simulink model "lvlh_control_sim"  (R2023b)
settings: Solver=ode5  StartTime=0.0  StopTime=100  RelTol=1e-3
values from neighbouring files (symbols this model uses):
  A = [ ... (first row only)    [complete_model.m]    (also in control_lvlh.m; lvlh_control.m = zeros(6,6); untitled.m = zeros(6,6))
  a = 6.851221970532768e+03    (= 6851.22197053)    [complete_model.m]    (also in control_lvlh.m; lvlh_control.m; untitled.m)
  alpha1 = 0.4    [complete_model.m]    (also in control_lvlh.m; lvlh_control.m; untitled.m)
  alpha2 = 0.1    [complete_model.m]    (also in control_lvlh.m; lvlh_control.m; untitled.m)
  alpha3 = 0.5    [complete_model.m]    (also in control_lvlh.m; lvlh_control.m; untitled.m)
  B = [ ... (first row only)    [complete_model.m]    (also in control_lvlh.m; lvlh_control.m = zeros(6,3); untitled.m = zeros(6,3))
  C = [ ... (first row only)    [complete_model.m]    (also in control_lvlh.m; lvlh_control.m = [[0 0 0 1 0 0];[0 0 0 0 1 0]; [0 0 0 0 0 1]]; untitled.m = [[0 0 0 1 0 0];[0 0 0 0 1 0]; [0 0 0 0 0 1]])
  D = zeros(3)    [complete_model.m]    (also in control_lvlh.m; lvlh_control.m = zeros(3,3); untitled.m = zeros(3,3))
  e = 0    [complete_model.m]    (also in control_lvlh.m; lvlh_control.m; untitled.m)
  FOV_earth = deg2rad(33)    [complete_model.m]    (also in control_lvlh.m; lvlh_control.m; untitled.m)
  FOV_sun = deg2rad(85)    [control_lvlh.m]    (also in lvlh_control.m; untitled.m)
  freq_earth = 30    [complete_model.m]    (also in control_lvlh.m = 5; lvlh_control.m = 5; untitled.m = 5)
  freq_mag = 30    [complete_model.m]    (also in control_lvlh.m = 5; lvlh_control.m = 5; untitled.m = 5)
  freq_sun = 30    [complete_model.m]    (also in control_lvlh.m = 5; lvlh_control.m = 5; untitled.m = 5)
  H0 = sqrt(g01^2+g11^2+h11^2)*1e-9    [complete_model.m]    (also in control_lvlh.m; lvlh_control.m; untitled.m)
  I = diag([I1 I2 I3])    [complete_model.m]    (also in control_lvlh.m; lvlh_control.m; untitled.m)
  Iinv = I\eye(3)    [complete_model.m]    (also in control_lvlh.m; lvlh_control.m; untitled.m)
  incl = deg2rad(11.5)    [complete_model.m]    (also in control_lvlh.m; lvlh_control.m; untitled.m)
  jb = [0.01; 0.05; 0.01]    [complete_model.m]    (also in control_lvlh.m; lvlh_control.m; untitled.m)
  K = place(A,B,p)    [complete_model.m]    (also in control_lvlh.m = [Kd Kp]; lvlh_control.m = 1/100*K)
  L = Ltr'    [lvlh_control.m]    (also in untitled.m)
  n = sqrt(mu/a^3)    [complete_model.m]    (also in control_lvlh.m; lvlh_control.m; untitled.m)
  omega0 = 0.06 * rand(3,1)    [complete_model.m]    (also in control_lvlh.m = [0; 0; n]; lvlh_control.m = [0; 0; n]; untitled.m = [0; 0; n])
  omegaE = deg2rad(15)/3600    [complete_model.m]    (also in control_lvlh.m; lvlh_control.m; untitled.m)
  rs = -rr    [complete_model.m]    (also in control_lvlh.m; lvlh_control.m; untitled.m)
  Rt = astroConstants(23)    [complete_model.m]    (also in control_lvlh.m; lvlh_control.m; untitled.m)
  s0 = 2*pi*rand(3,1)    [complete_model.m]    (also in control_lvlh.m = [2.099, -0.2003, -1.703]; lvlh_control.m = [2.099, -0.2003, -1.703]; untitled.m = [2.099, -0.2003, -1.703])
  tol = 0.2    [complete_model.m]    (also in control_lvlh.m; lvlh_control.m; untitled.m)
  variance_E_sens = (deg2rad(0.05)/3)^2    [lvlh_control.m]    (also in untitled.m)
undefined symbols (not defined in the file or in its folder): magnitude
libraries: vrlib x8, matrix_library x6, simulink x6, sharedutil x2, dspmathops x2, dspfactors x1, simulink_extras x1
(part 1 of 2)
settings Model: Creator=danie  LastModifiedBy=danie

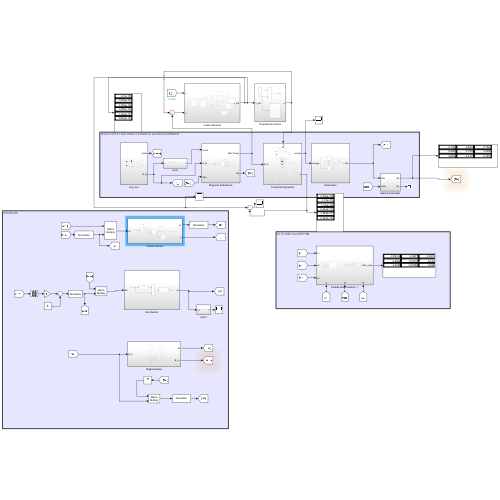
[thumbnail: Simulink's stored preview of the top-level diagram]
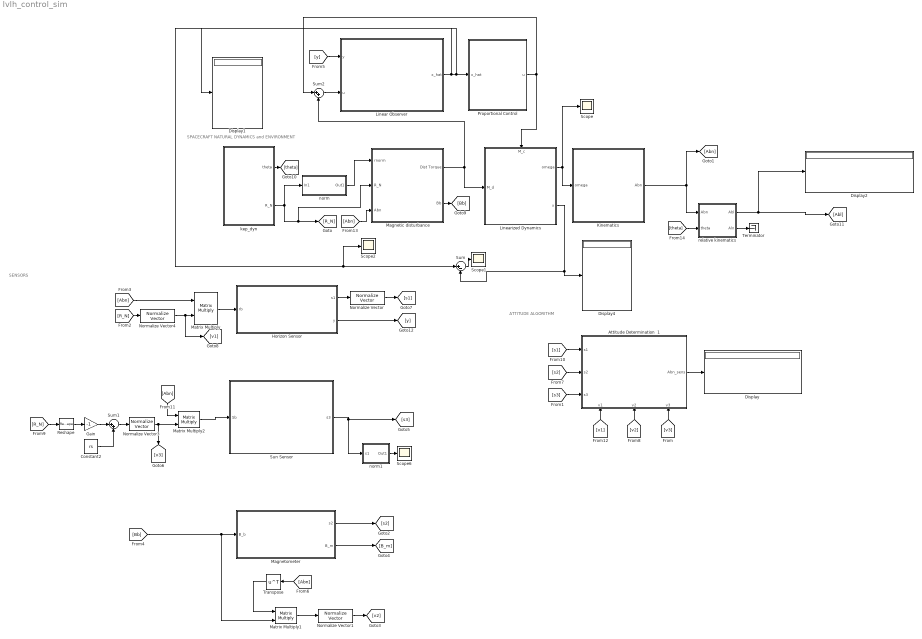
== system lvlh_control_sim ==
  note: SENSORS
  note: ATTITUDE ALGORITHM
  note: SPACECRAFT NATURAL DYNAMICS and ENVIRONMENT
  Attitude Determination  1 : Subsystem
      settings: PortSchema="{\"entries\":[{\"content\":{\"sides\":[{\"content\":{\"connectorIds\":[\"In1\",\"In2\",\"In3\"]},\"type\":\"ConnectorPlacement.EquallySpacedRectSide\",\"uuid\":\"730966cf-d0d7-44a0-92f0-b5324480e7cc\"},{\"content\":{\"connectorIds\":[\"Out1\"],\"side\":\"RIGHT\"},\"type\":\"ConnectorPlacement.EquallySpacedRectSide\",\"uuid\":\"c83e6b57-46fe-4a45-9824-d3495e15bf6a\"},{\"content\":{\"side\":\"TOP\"},\"type\":\"ConnectorPlacement.EquallySpacedRectSide\",\"uuid\":\"4938c298-c2b3-45b7-bcb0-70b8132dabc6\"},{\"content\":{\"connectorIds\":[\"In4\",\"In5\",\"In6\"],\"side\":\"BOTTOM\"},\"type\":\"ConnectorPlacement.EquallySpacedRectSide\",\"uuid\":\"6d6a244e-80db-423b-a0a5-9a5face48fcb\"}]},\"type\":\"ConnectorPlacement.EquallySpacedConnector\",\"uuid\":\"7eb6767d-3ff0-4577-86c9-ebc5e763f220\"}],\"packageUris\":[\"http://schema.mathworks.com/mf0/Connector/R2020b\"],\"version\":\"1.0\"}"
  Constant2 : Constant  Value=rs
  Display{,1..2,4} (4 alike) : Display
  Gain : Gain  Gain=-1
  Horizon Sensor : Subsystem
  Kinematics : Subsystem
  Linear Observer : Subsystem
  Linearized Dynamics : Subsystem
      settings: PortSchema="{\"entries\":[{\"content\":{\"sides\":[{\"content\":{\"connectorIds\":[\"In1\"]},\"type\":\"ConnectorPlacement.EquallySpacedRectSide\",\"uuid\":\"c1c0c392-5a65-42dc-acc1-f79aac47fb4a\"},{\"content\":{\"connectorIds\":[\"Out1\",\"Out2\"],\"side\":\"RIGHT\"},\"type\":\"ConnectorPlacement.EquallySpacedRectSide\",\"uuid\":\"022a04b8-112e-4b43-aa4b-234ec6f248c8\"},{\"content\":{\"connectorIds\":[\"In2\"],\"side\":\"TOP\"},\"type\":\"ConnectorPlacement.EquallySpacedRectSide\",\"uuid\":\"afc410f0-4ae5-435d-a431-df883452497d\"}]},\"type\":\"ConnectorPlacement.EquallySpacedConnector\",\"uuid\":\"3545f0ca-e723-442b-9659-f094d9054fb0\"}],\"packageUris\":[\"http://schema.mathworks.com/mf0/Connector/R2020b\"],\"version\":\"1.0\"}"
  Magnetic disturbance : Subsystem
  Magnetometer : Subsystem
  Matrix Multiply : Product  Multiplication=Matrix(*)
  Matrix Multiply1 : Product  Multiplication=Matrix(*)
  Matrix Multiply2 : Product  Multiplication=Matrix(*)
  Normalize Vector{,1,3..4} (4 alike) : vrlib/Utilities/Normalize Vector  maxzero=0
  Proportional Control : Subsystem
  Reshape : Reshape  OutputDimensionality=Column vector (2-D)
  Scope{,1..2,6} (4 alike) : Scope
  Sum : Sum  Inputs=|+-
  Sum1 : Sum  Inputs=|++
  Sum2 : Sum  Inputs=|++
  Sun Sensor : Subsystem
  Terminator : Terminator
  Transpose : Math  Operator=transpose
  kep_dyn : Subsystem
  norm : Subsystem
  norm1 : Subsystem
  relative kinematics : Subsystem
  wires:
  Kinematics/1(Abn) -> relative kinematics/1(Abn), [Abn]
  [v1] -> Attitude Determination  1/4(v1)
  [Abn] -> Matrix Multiply2/1
  [theta] -> relative kinematics/2(theta)
  Matrix Multiply/1 -> Horizon Sensor/1(rb)
  relative kinematics/1(Abl) -> Display2/1, [Abl]
  Matrix Multiply1/1 -> Normalize Vector1/1
  norm/1(Out1) -> Magnetic disturbance/1(rnorm)
  Normalize Vector1/1 -> [v2]
  [s2] -> Attitude Determination  1/2(s2)
  Constant2/1 -> Sum1/2
  Sum1/1 -> Normalize Vector3/1
  Normalize Vector/1 -> [s1]
  [s1] -> Attitude Determination  1/1(s1)
  kep_dyn/1(theta) -> [theta]
  kep_dyn/2(R_N) -> Magnetic disturbance/2(R_N), [R_N], norm/1(In1)
  [s3] -> Attitude Determination  1/3(s3)
  Magnetometer/2("B_m ") -> [B_m]
  [Abn] -> Transpose/1
  Magnetic disturbance/2(Bb) -> [Bb]
  [Abn] -> Magnetic disturbance/3(Abn)
  Horizon Sensor/1(s1) -> Normalize Vector/1
  [R_N] -> Normalize Vector4/1
  [Bb] -> Matrix Multiply1/2, Magnetometer/1(B_b)
  Sun Sensor/1(s3) -> norm1/1(s1), [s3]
  [R_N] -> Reshape/1
  Matrix Multiply2/1 -> Sun Sensor/1(Sb)
  Transpose/1 -> Matrix Multiply1/1
  Normalize Vector4/1 -> [v1], Matrix Multiply/2
  norm1/1(Out1) -> Scope6/1
  Attitude Determination  1/1(Abn_sens) -> Display/1
  Normalize Vector3/1 -> Matrix Multiply2/2, [v3]
  Magnetometer/1(s2) -> [s2]
  [v3] -> Attitude Determination  1/6(v3)
  relative kinematics/2(Aln) -> Terminator/1
  [Abn] -> Matrix Multiply/1
  Gain/1 -> Sum1/1
  [v2] -> Attitude Determination  1/5(v2)
  Reshape/1 -> Gain/1
  Magnetic disturbance/1(Dist Torque) -> Sum2/2, Linearized Dynamics/1(M_d)
  Linearized Dynamics/1(omega) -> Kinematics/1(omega), Scope/1
  Horizon Sensor/2(y) -> [y]
  [y] -> Linear Observer/1(y)
  Linearized Dynamics/2(x) -> Sum/2, Display4/1
  Sum/1 -> Scope1/1
  Linear Observer/1(x_hat) -> Display1/1, Scope2/1, Sum/1, Proportional Control/1(x_hat)
  Sum2/1 -> Linear Observer/2(u)
  Proportional Control/1(u) -> Linearized Dynamics/2(M_c), Sum2/1

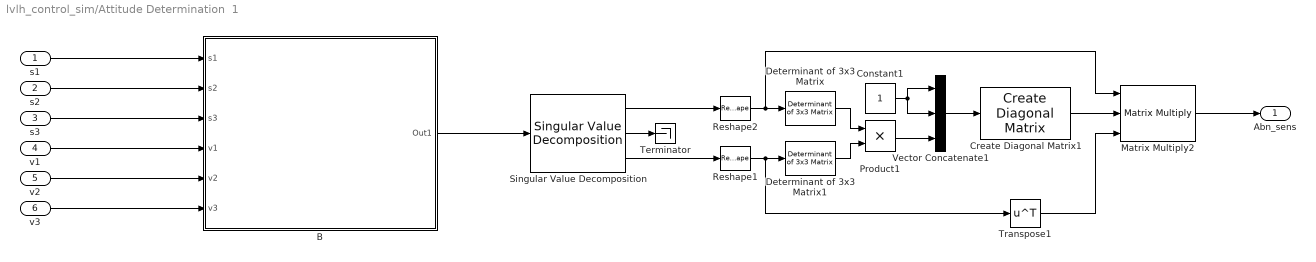
== system lvlh_control_sim/Attitude Determination  1 ==
  s1 : Inport
  s2 : Inport  Port=2
  s3 : Inport  Port=3
  v1 : Inport  Port=4
  v2 : Inport  Port=5
  v3 : Inport  Port=6
  B : Subsystem
  Constant1 : Constant
  Create Diagonal Matrix1 : matrix_library/Create Diagonal Matrix
      settings: LibrarySourceBlock=|
      | simulink/Matrix
      | Operations/Create Diagonal
      | Matrix
  Determinant of 3x3 Matrix : sharedutil/Determinant of 3x3 Matrix  aMode=aMode
      settings: LibrarySourceBlock=|
      | aerolibutil/Determinant of
      | 3x3 Matrix
  Determinant of 3x3 Matrix1 : sharedutil/Determinant of 3x3 Matrix  aMode=aMode
      settings: LibrarySourceBlock=|
      | aerolibutil/Determinant of
      | 3x3 Matrix
  Matrix Multiply2 : Product  Inputs=3  Multiplication=Matrix(*)
  Product1 : Product
  Reshape1 : Reshape  OutputDimensionality=Customize  OutputDimensions=[3,3]
  Reshape2 : Reshape  OutputDimensionality=Customize  OutputDimensions=[3,3]
  Singular Value Decomposition : dspfactors/Singular Value Decomposition  wantv=on  wanterr=off  SimulateUsing=Interpreted execution
  Terminator : Terminator
  Transpose1 : Math  Operator=transpose
  Vector Concatenate1 : Concatenate  NumInputs=3
  Abn_sens : Outport
  wires:
  Reshape1/1 -> Transpose1/1, Determinant of 3x3 Matrix1/1
  Singular Value Decomposition/3 -> Reshape1/1
  Singular Value Decomposition/1 -> Reshape2/1
  Reshape2/1 -> Determinant of 3x3 Matrix/1, Matrix Multiply2/1
  Determinant of 3x3 Matrix1/1 -> Product1/2
  Determinant of 3x3 Matrix/1 -> Product1/1
  Product1/1 -> Vector Concatenate1/3
  Constant1/1 -> Vector Concatenate1/2, Vector Concatenate1/1
  Vector Concatenate1/1 -> Create Diagonal Matrix1/1
  Create Diagonal Matrix1/1 -> Matrix Multiply2/2
  Transpose1/1 -> Matrix Multiply2/3
  s1/1 -> B/1(s1)
  s2/1 -> B/2(s2)
  s3/1 -> B/3(s3)
  v1/1 -> B/4(v1)
  v2/1 -> B/5(v2)
  v3/1 -> B/6(v3)
  B/1(Out1) -> Singular Value Decomposition/1
  Matrix Multiply2/1 -> Abn_sens/1
  Singular Value Decomposition/2 -> Terminator/1

== system lvlh_control_sim/Horizon Sensor ==
  rb : Inport
  Constant : Constant
  Display : Display
  Display1 : Display
  EH sensor modeling : Subsystem
  FOV CHECK : Subsystem  Commented=on
  Gain : Gain  Gain=-1
  Product1 : Product
  s1 : Outport
  y : Outport  Port=2
  wires:
  rb/1 -> Gain/1
  Product1/1 -> EH sensor modeling/1(rb)
  EH sensor modeling/1(q) -> s1/1  "direction of earth"
  EH sensor modeling/2(y) -> y/1, Display/1
  Gain/1 -> FOV CHECK/1(In1), Display1/1, Product1/2
  Constant/1 -> Product1/1

== system lvlh_control_sim/Kinematics ==
  omega : Inport
  Kinematics 312 : Subsystem
  Kinematics 313 : Subsystem
  Merge : Merge
  NOT : Logic  Operator=NOT  IconShape=distinctive  AllPortsSameDT=off  OutDataTypeStr=boolean
  System switcher : Subsystem
  To Workspace : ToWorkspace  VariableName=A  SaveFormat=Timeseries  SampleTime=-1
  Abn : Outport
  wires:
  NOT/1 -> Kinematics 313/Enable
  omega/1 -> Kinematics 312/1(w), Kinematics 313/1(w)
  System switcher/1(flag) -> Kinematics 312/Enable, NOT/1
  Kinematics 313/1(A) -> Merge/2
  Merge/1 -> Abn/1, To Workspace/1  "A"
  Kinematics 312/1(A) -> Merge/1

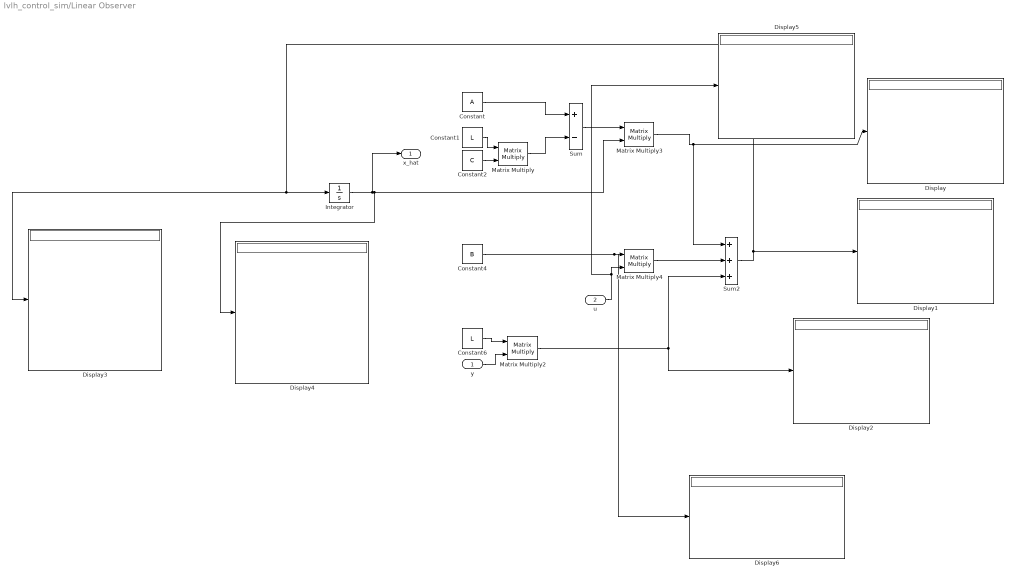
== system lvlh_control_sim/Linear Observer ==
  y : Inport
  u : Inport  Port=2
  Constant : Constant  Value=A
  Constant1 : Constant  Value=L
  Constant2 : Constant  Value=C
  Constant4 : Constant  Value=B
  Constant6 : Constant  Value=L
  Display{,1..6} (7 alike) : Display
  Integrator : Integrator  InitialCondition=[0;0;0;0;0;0]
  Matrix Multiply{,2..4} (4 alike) : Product  Multiplication=Matrix(*)
  Sum : Sum  Inputs=+-
  Sum2 : Sum  Inputs=+++
  x_hat : Outport
  wires:
  Constant1/1 -> Matrix Multiply/1
  Constant2/1 -> Matrix Multiply/2
  Matrix Multiply/1 -> Sum/2
  Constant/1 -> Sum/1
  Constant6/1 -> Matrix Multiply2/1
  y/1 -> Matrix Multiply2/2
  u/1 -> Matrix Multiply4/2, Display5/1
  Constant4/1 -> Display6/1, Matrix Multiply4/1
  Sum/1 -> Matrix Multiply3/1
  Matrix Multiply4/1 -> Sum2/2
  Matrix Multiply2/1 -> Sum2/3, Display2/1
  Matrix Multiply3/1 -> Display/1, Sum2/1
  Sum2/1 -> Integrator/1, Display3/1, Display1/1
  Integrator/1 -> Display4/1, Matrix Multiply3/2, x_hat/1

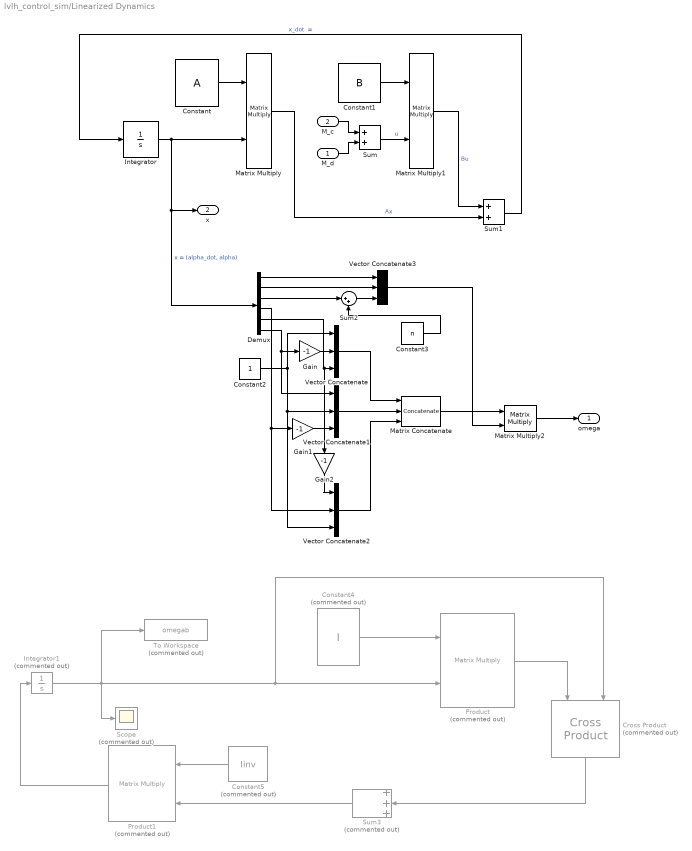
== system lvlh_control_sim/Linearized Dynamics ==
  M_d : Inport
  M_c : Inport  Port=2
  Constant : Constant  Value=A
  Constant1 : Constant  Value=B
  Constant2 : Constant
  Constant3 : Constant  Value=n
  Constant4 : Constant  Commented=on  Value=I
  Constant5 : Constant  Commented=on  Value=Iinv
  Cross Product : matrix_library/Cross Product  Commented=on
  Demux : Demux  Outputs=6
  Gain : Gain  Gain=-1
  Gain1 : Gain  Gain=-1
  Gain2 : Gain  Gain=-1
  Integrator : Integrator  InitialCondition=[1e-6; 1e-6; n; 0;0;0]
  Integrator1 : Integrator  Commented=on  InitialCondition=omega0
  Matrix Concatenate : Concatenate  NumInputs=3  Mode=Multidimensional array  ConcatenateDimension=2
  Matrix Multiply : Product  Multiplication=Matrix(*)
  Matrix Multiply1 : Product  Multiplication=Matrix(*)
  Matrix Multiply2 : Product  Multiplication=Matrix(*)
  Product : Product  Commented=on  Multiplication=Matrix(*)
  Product1 : Product  Commented=on  Multiplication=Matrix(*)
  Scope : Scope  Commented=on
  Sum : Sum
  Sum1 : Sum
  Sum2 : Sum  Inputs=|++
  Sum3 : Sum  Commented=on  Inputs=+++
  To Workspace : ToWorkspace  Commented=on  VariableName=omegab  SampleTime=-1
  Vector Concatenate{,1..3} (4 alike) : Concatenate  NumInputs=3
  omega : Outport
  x : Outport  Port=2
  wires:
  Integrator/1 -> x/1, Demux/1, Matrix Multiply/2  "x = (alpha_dot, alpha)"
  Constant/1 -> Matrix Multiply/1
  Constant1/1 -> Matrix Multiply1/1
  Sum/1 -> Matrix Multiply1/2  "u"
  M_c/1 -> Sum/1
  Matrix Multiply1/1 -> Sum1/1  "Bu"
  Matrix Multiply/1 -> Sum1/2  "Ax"
  Sum1/1 -> Integrator/1  "x_dot  ="
  Constant2/1 -> Vector Concatenate/1, Vector Concatenate2/3, Vector Concatenate1/2
  Demux/6 -> Vector Concatenate1/1, Gain/1
  Gain/1 -> Vector Concatenate/2
  Demux/5 -> Vector Concatenate/3, Gain2/1
  Demux/4 -> Vector Concatenate2/2, Gain1/1
  Gain1/1 -> Vector Concatenate1/3
  Gain2/1 -> Vector Concatenate2/1
  Vector Concatenate/1 -> Matrix Concatenate/1
  Vector Concatenate1/1 -> Matrix Concatenate/2
  Vector Concatenate2/1 -> Matrix Concatenate/3
  Matrix Concatenate/1 -> Matrix Multiply2/1
  Demux/1 -> Vector Concatenate3/1
  Demux/2 -> Vector Concatenate3/2
  Demux/3 -> Sum2/1
  Constant3/1 -> Sum2/2
  Sum2/1 -> Vector Concatenate3/3
  Vector Concatenate3/1 -> Matrix Multiply2/2
  Matrix Multiply2/1 -> omega/1
  Sum3/1 -> Product1/2
  Constant4/1 -> Product/1
  Constant5/1 -> Product1/1
  Cross Product/1 -> Sum3/2
  Integrator1/1 -> To Workspace/1, Scope/1, Product/2, Cross Product/2
  Product/1 -> Cross Product/1
  Product1/1 -> Integrator1/1
  M_d/1 -> Sum/2

== system lvlh_control_sim/Magnetic disturbance ==
  rnorm : Inport
  R_N : Inport  Port=2
  Abn : Inport  Port=3
  "Magnetic Torque " : Subsystem
  Matrix Multiply : Product  Multiplication=Matrix(*)
  Normalize Vector : vrlib/Utilities/Normalize Vector  maxzero=0
  Scope : Scope
  Scope1 : Scope
  To Workspace1 : ToWorkspace  VariableName=mag_torque  SampleTime=-1
  Dist Torque : Outport
  Bb : Outport  Port=2
  wires:
  rnorm/1 -> "Magnetic Torque "/1(rnorm)
  Abn/1 -> Matrix Multiply/1, "Magnetic Torque "/2(Abn)
  "Magnetic Torque "/1(M_mag) -> To Workspace1/1, Scope1/1, Dist Torque/1
  "Magnetic Torque "/2(Bb) -> Scope/1, Bb/1
  R_N/1 -> Normalize Vector/1
  Matrix Multiply/1 -> "Magnetic Torque "/3(rb)
  Normalize Vector/1 -> Matrix Multiply/2

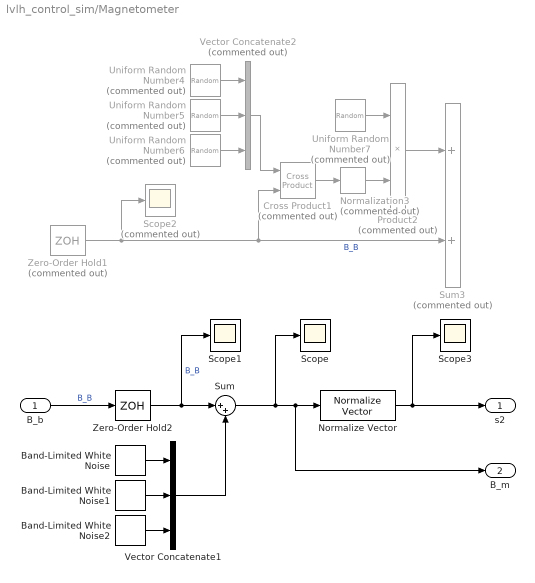
== system lvlh_control_sim/Magnetometer ==
  B_b : Inport
  Band-Limited White Noise : simulink/Sources/Band-Limited White Noise  Cov=[1.18^2 *1e-18]  Ts=1/freq_mag  seed=[23341]
  Band-Limited White Noise1 : simulink/Sources/Band-Limited White Noise  Cov=[1.18^2 *1e-18]  Ts=1/freq_mag  seed=[23341]
  Band-Limited White Noise2 : simulink/Sources/Band-Limited White Noise  Cov=[1.18^2 *1e-18]  Ts=1/freq_mag  seed=[23341]
  Cross Product1 : matrix_library/Cross Product  Commented=on
  Normalization3 : dspmathops/Normalization  Commented=on  NormType=2-norm  Bias=1e-10  NormOver=Each column  Dimension=1  roundingMode=Floor  overflowMode=off  accumDataTypeStr=Inherit: Same as product output  accumLastDataTypeStr=Inherit: Same as product output  outputDataTypeStr=Inherit: Same as product output  outputMin=[]  outputMax=[]  outputLastDataTypeStr=Inherit: Same as product output
  Normalize Vector : vrlib/Utilities/Normalize Vector  maxzero=0
  Product2 : Product  Commented=on
  Scope : Scope
  Scope1 : Scope
  Scope2 : Scope  Commented=on
  Scope3 : Scope
  Sum : Sum  Inputs=|++
  Sum3 : Sum  Commented=on
  Uniform Random Number4 : UniformRandomNumber  Commented=on  SampleTime=1/30
  Uniform Random Number5 : UniformRandomNumber  Commented=on  SampleTime=1/30
  Uniform Random Number6 : UniformRandomNumber  Commented=on  SampleTime=1/30
  Uniform Random Number7 : UniformRandomNumber  Commented=on  Minimum=0  Maximum=tan(deg2rad(0.5))  SampleTime=1/30
  Vector Concatenate1 : Concatenate  NumInputs=3
  Vector Concatenate2 : Concatenate  Commented=on  NumInputs=3
  Zero-Order Hold1 : ZeroOrderHold  Commented=on  SampleTime=1/30
  Zero-Order Hold2 : ZeroOrderHold  SampleTime=1/freq_mag
  s2 : Outport
  "B_m " : Outport  Port=2
  wires:
  Zero-Order Hold1/1 -> Cross Product1/2, Sum3/2, Scope2/1  "B_B"
  Product2/1 -> Sum3/1
  Normalization3/1 -> Product2/2
  Uniform Random Number4/1 -> Vector Concatenate2/1
  Uniform Random Number6/1 -> Vector Concatenate2/3
  Vector Concatenate2/1 -> Cross Product1/1
  Cross Product1/1 -> Normalization3/1
  Uniform Random Number5/1 -> Vector Concatenate2/2
  Uniform Random Number7/1 -> Product2/1
  B_b/1 -> Zero-Order Hold2/1  "B_B"
  Zero-Order Hold2/1 -> Scope1/1, Sum/1  "B_B"
  Band-Limited White Noise2/1 -> Vector Concatenate1/3
  Band-Limited White Noise1/1 -> Vector Concatenate1/2
  Band-Limited White Noise/1 -> Vector Concatenate1/1
  Normalize Vector/1 -> Scope3/1, s2/1
  Vector Concatenate1/1 -> Sum/2
  Sum/1 -> Scope/1, "B_m "/1, Normalize Vector/1

== system lvlh_control_sim/Proportional Control ==
  x_hat : Inport
  Constant : Constant  Value=-K
  Display : Display
  Matrix Multiply : Product  Multiplication=Matrix(*)
  u : Outport
  wires:
  x_hat/1 -> Display/1, Matrix Multiply/2
  Constant/1 -> Matrix Multiply/1
  Matrix Multiply/1 -> u/1

== system lvlh_control_sim/Sun Sensor ==
  Sb : Inport
  FOV CHECK : Subsystem
  Product : Product
  Sun Sensor Modeling : Subsystem
  s3 : Outport
  wires:
  Sb/1 -> Product/2, FOV CHECK/1(In1)  "Sb"
  Sun Sensor Modeling/1(s3) -> s3/1
  Product/1 -> Sun Sensor Modeling/1(Sb)  "Sb"
  FOV CHECK/1(b) -> Product/1

== system lvlh_control_sim/kep_dyn ==
  A_np : Constant  Value=A_pn'
  Constant : Constant  Value=0
  Constant1 : Constant  Value=e
  Cos : Trigonometry  Operator=cos
  Integrator : Integrator
  Matrix Multiply : Product  Multiplication=Matrix(*)
  Product2 : Product
  Sin : Trigonometry
  Vector Concatenate : Concatenate  NumInputs=3
  r_norm : Subsystem
  theta integration : Subsystem
      settings: PortSchema="{\"entries\":[{\"content\":{\"sides\":[{\"content\":{\"connectorIds\":[\"In1\"]},\"type\":\"ConnectorPlacement.EquallySpacedRectSide\",\"uuid\":\"3f1b1ec9-07ed-4eb1-9e41-630dc5613e97\"},{\"content\":{\"connectorIds\":[\"Out1\",\"In2\"],\"side\":\"RIGHT\"},\"type\":\"ConnectorPlacement.EquallySpacedRectSide\",\"uuid\":\"22d0f7bc-714c-4365-a26c-07047ff4be14\"},{\"content\":{\"side\":\"TOP\"},\"type\":\"ConnectorPlacement.EquallySpacedRectSide\",\"uuid\":\"875f7006-d698-4730-93ae-1a7d05f24054\"}]},\"type\":\"ConnectorPlacement.EquallySpacedConnector\",\"uuid\":\"799b65b1-faea-432b-9f3f-2d21984184cd\"}],\"packageUris\":[\"http://schema.mathworks.com/mf0/Connector/R2020b\"],\"version\":\"1.0\"}"
  theta : Outport
  R_N : Outport  Port=2
  wires:
  Integrator/1 -> Sin/1, Cos/1, r_norm/2(theta), theta/1, theta integration/1(theta)
  theta integration/1(theta_dot) -> Integrator/1
  Constant/1 -> Vector Concatenate/3
  Cos/1 -> Vector Concatenate/1
  Constant1/1 -> r_norm/1(e), theta integration/2(e)
  r_norm/1(r) -> Product2/1
  Vector Concatenate/1 -> Product2/2
  Sin/1 -> Vector Concatenate/2
  A_np/1 -> Matrix Multiply/1
  Product2/1 -> Matrix Multiply/2
  Matrix Multiply/1 -> R_N/1

== system lvlh_control_sim/norm ==
  In1 : Inport
  Dot Product : DotProduct  OutDataTypeStr=Inherit: Inherit via internal rule
  Sqrt : Sqrt
  Out1 : Outport
  wires:
  In1/1 -> Dot Product/1, Dot Product/2
  Dot Product/1 -> Sqrt/1
  Sqrt/1 -> Out1/1

== system lvlh_control_sim/norm1 ==
  s1 : Inport
  Dot Product : DotProduct  OutDataTypeStr=Inherit: Inherit via internal rule
  Square Root : Sqrt
  Out1 : Outport
  wires:
  s1/1 -> Dot Product/1, Dot Product/2
  Dot Product/1 -> Square Root/1
  Square Root/1 -> Out1/1

== system lvlh_control_sim/relative kinematics ==
  Abn : Inport
  theta : Inport  Port=2
  Constant : Constant  Value=A_pn'
  Matrix Multiply : Product  Multiplication=Matrix(*)
  Matrix Multiply2 : Product  Multiplication=Matrix(*)
  Subsystem : Subsystem
  Transpose : Math  Operator=transpose
  Abl : Outport
  Aln : Outport  Port=2
  wires:
  Abn/1 -> Matrix Multiply2/1
  Matrix Multiply/1 -> Transpose/1, Matrix Multiply2/2  "A_nl"
  Matrix Multiply2/1 -> Abl/1
  theta/1 -> Subsystem/1(theta)
  Subsystem/1(A_PL) -> Matrix Multiply/2  "A_PL"
  Constant/1 -> Matrix Multiply/1  "A_np"
  Transpose/1 -> Aln/1

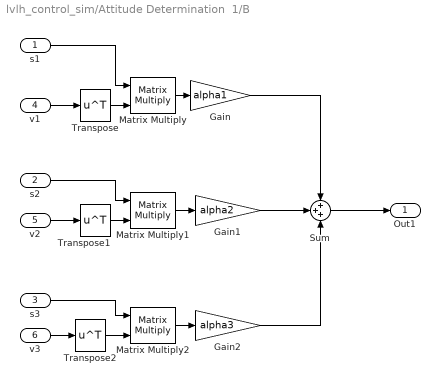
== system lvlh_control_sim/Attitude Determination  1/B ==
  s1 : Inport
  s2 : Inport  Port=2
  s3 : Inport  Port=3
  v1 : Inport  Port=4
  v2 : Inport  Port=5
  v3 : Inport  Port=6
  Gain : Gain  Gain=alpha1
  Gain1 : Gain  Gain=alpha2
  Gain2 : Gain  Gain=alpha3
  Matrix Multiply : Product  Multiplication=Matrix(*)
  Matrix Multiply1 : Product  Multiplication=Matrix(*)
  Matrix Multiply2 : Product  Multiplication=Matrix(*)
  Sum : Sum  Inputs=+++
  Transpose : Math  Operator=transpose
  Transpose1 : Math  Operator=transpose
  Transpose2 : Math  Operator=transpose
  Out1 : Outport
  wires:
  v1/1 -> Transpose/1
  Transpose/1 -> Matrix Multiply/2
  s1/1 -> Matrix Multiply/1
  Transpose1/1 -> Matrix Multiply1/2
  s2/1 -> Matrix Multiply1/1
  Transpose2/1 -> Matrix Multiply2/2
  v3/1 -> Transpose2/1
  Sum/1 -> Out1/1
  Matrix Multiply/1 -> Gain/1
  Matrix Multiply1/1 -> Gain1/1
  Matrix Multiply2/1 -> Gain2/1
  Gain/1 -> Sum/1
  Gain1/1 -> Sum/2
  Gain2/1 -> Sum/3
  v2/1 -> Transpose1/1
  s3/1 -> Matrix Multiply2/1

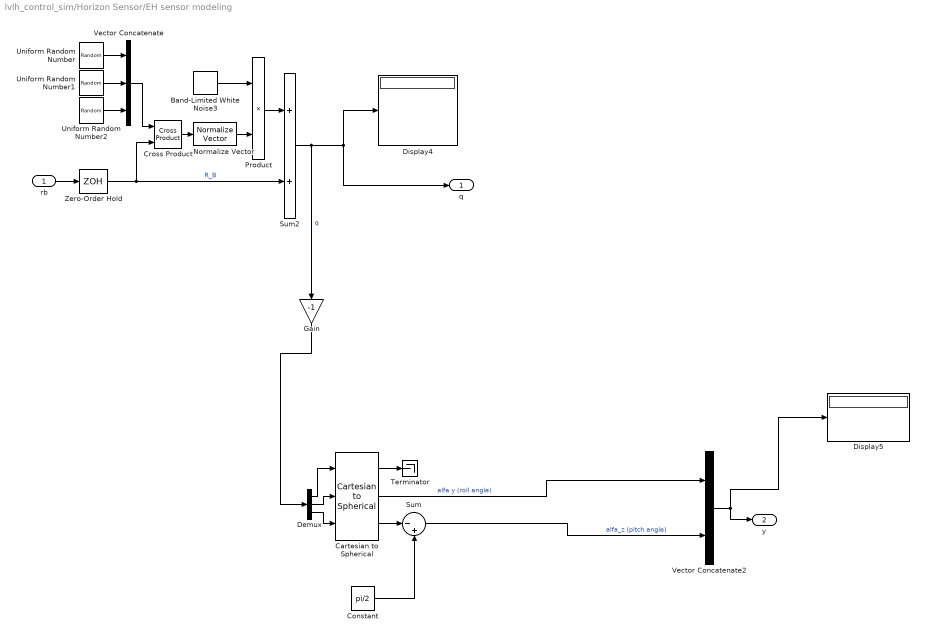
== system lvlh_control_sim/Horizon Sensor/EH sensor modeling ==
  rb : Inport
  Band-Limited White Noise3 : simulink/Sources/Band-Limited White Noise  Cov=[variance_E_sens*1/freq_earth]  Ts=1/freq_earth  seed=[23341]
  Cartesian to Spherical : simulink_extras/Transformations/Cartesian to Spherical
  Constant : Constant  Value=pi/2
  Cross Product : matrix_library/Cross Product
  Demux : Demux  Outputs=3
  Display4 : Display
  Display5 : Display
  Gain : Gain  Gain=-1
  Normalize Vector : vrlib/Utilities/Normalize Vector  maxzero=0
  Product : Product
  Sum : Sum  Inputs=|-+
  Sum2 : Sum
  Terminator : Terminator
  Uniform Random Number : UniformRandomNumber  SampleTime=0.1
  Uniform Random Number1 : UniformRandomNumber  SampleTime=0.1
  Uniform Random Number2 : UniformRandomNumber  SampleTime=0.1
  Vector Concatenate : Concatenate  NumInputs=3
  Vector Concatenate2 : Concatenate
  Zero-Order Hold : ZeroOrderHold  SampleTime=1/freq_earth
  q : Outport
  y : Outport  Port=2
  wires:
  Product/1 -> Sum2/1
  Band-Limited White Noise3/1 -> Product/1
  Uniform Random Number1/1 -> Vector Concatenate/2
  Uniform Random Number2/1 -> Vector Concatenate/3
  Normalize Vector/1 -> Product/2
  Uniform Random Number/1 -> Vector Concatenate/1
  Zero-Order Hold/1 -> Cross Product/2, Sum2/2  "R_B"
  Vector Concatenate/1 -> Cross Product/1
  Cross Product/1 -> Normalize Vector/1
  Sum2/1 -> Display4/1, q/1, Gain/1  "q"
  rb/1 -> Zero-Order Hold/1
  Demux/1 -> Cartesian to Spherical/1
  Demux/2 -> Cartesian to Spherical/2
  Demux/3 -> Cartesian to Spherical/3
  Cartesian to Spherical/1 -> Terminator/1
  Cartesian to Spherical/2 -> Vector Concatenate2/1  "alfa y (roll angle)"
  Vector Concatenate2/1 -> y/1, Display5/1
  Cartesian to Spherical/3 -> Sum/1
  Sum/1 -> Vector Concatenate2/2  "alfa_z (pitch angle)"
  Constant/1 -> Sum/2
  Gain/1 -> Demux/1

== system lvlh_control_sim/Horizon Sensor/FOV CHECK ==
  In1 : Inport
  Acos : Trigonometry  Operator=acos
  Dot Product : DotProduct  OutDataTypeStr=Inherit: Inherit via internal rule
  FOV angle : Constant  Value=FOV_earth
  Less Than : RelationalOperator  Operator=<  OutDataTypeStr=boolean  RndMeth=Simplest  InputSameDT=off
  optical axis : Constant  Value=[-1;0;0]
  b : Outport
  wires:
  optical axis/1 -> Dot Product/1
  In1/1 -> Dot Product/2
  Dot Product/1 -> Acos/1
  FOV angle/1 -> Less Than/2
  Acos/1 -> Less Than/1
  Less Than/1 -> b/1

== system lvlh_control_sim/Kinematics/Kinematics 312 ==
  w : Inport
  Enable : EnablePort  StatesWhenEnabling=reset
  A - s_312 : Subsystem
  Display : Display
  Display1 : Display
  Euler angles : Subsystem
  IC : InitialCondition  Value=s0
  s_312 - A : Subsystem
  s_313 - A : Subsystem
  A : Outport
  wires:
  s_312 - A/1(A) -> Display1/1, A/1  "A"
  Euler angles/1(s) -> s_312 - A/1(s)  "s"
  w/1 -> Euler angles/1(w)
  IC/1 -> Display/1, Euler angles/2(s0)
  A - s_312/1(s) -> IC/1
  s_313 - A/1(A) -> A - s_312/1(A)
  [s_313] -> s_313 - A/1(s)

== system lvlh_control_sim/Kinematics/Kinematics 313 ==
  w : Inport
  Enable : EnablePort  StatesWhenEnabling=reset
  A - s_313 : Subsystem
  Euler angles : Subsystem
  s_312 - A : Subsystem
  s_313 - A : Subsystem
  A : Outport
  wires:
  w/1 -> Euler angles/1(w)
  Euler angles/1(s) -> s_313 - A/1(s)
  s_313 - A/1(A) -> A/1
  A - s_313/1(s) -> Euler angles/2(s0)
  s_312 - A/1(A) -> A - s_313/1(A)
  [s_312] -> s_312 - A/1(s)

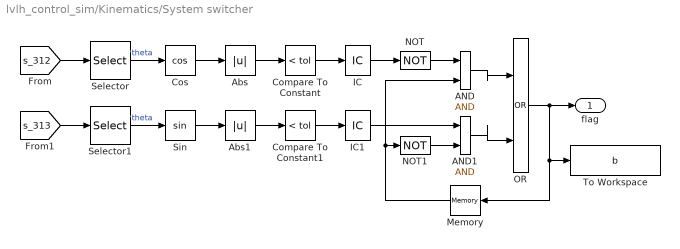
== system lvlh_control_sim/Kinematics/System switcher ==
  AND : Logic  IconShape=distinctive  AllPortsSameDT=off  OutDataTypeStr=boolean
  AND1 : Logic  IconShape=distinctive  AllPortsSameDT=off  OutDataTypeStr=boolean
  Abs : Abs  SaturateOnIntegerOverflow=off
  Abs1 : Abs  SaturateOnIntegerOverflow=off
  Compare To Constant : simulink/Logic and Bit Operations/Compare To Constant  relop=<  const=tol  OutDataTypeStr=boolean
  Compare To Constant1 : simulink/Logic and Bit Operations/Compare To Constant  relop=<  const=tol  OutDataTypeStr=boolean
  Cos : Trigonometry  Operator=cos
  IC : InitialCondition  Value=0
  IC1 : InitialCondition  Value=0
  Memory : Memory  InitialCondition=1
  NOT : Logic  Operator=NOT  IconShape=distinctive  AllPortsSameDT=off  OutDataTypeStr=boolean
  NOT1 : Logic  Operator=NOT  IconShape=distinctive  AllPortsSameDT=off  OutDataTypeStr=boolean
  OR : Logic  Operator=OR  IconShape=distinctive  AllPortsSameDT=off  OutDataTypeStr=boolean
  Selector : Selector  InputPortWidth=3  IndexOptions=Index vector (dialog)  Indices=2  OutputSizes=1
  Selector1 : Selector  InputPortWidth=3  IndexOptions=Index vector (dialog)  Indices=2  OutputSizes=1
  Sin : Trigonometry
  To Workspace : ToWorkspace  VariableName=b  SaveFormat=Timeseries  SampleTime=-1
  flag : Outport
  wires:
  Cos/1 -> Abs/1
  [s_312] -> Selector/1
  Compare To Constant/1 -> IC/1
  Selector1/1 -> Sin/1  "theta"
  Abs/1 -> Compare To Constant/1
  Compare To Constant1/1 -> IC1/1
  Selector/1 -> Cos/1  "theta"
  Abs1/1 -> Compare To Constant1/1
  Sin/1 -> Abs1/1
  [s_313] -> Selector1/1
  IC/1 -> NOT/1
  NOT/1 -> AND/1
  AND/1 -> OR/1
  NOT1/1 -> AND1/2
  IC1/1 -> AND1/1
  AND1/1 -> OR/2
  OR/1 -> To Workspace/1, Memory/1, flag/1
  Memory/1 -> AND/2, NOT1/1

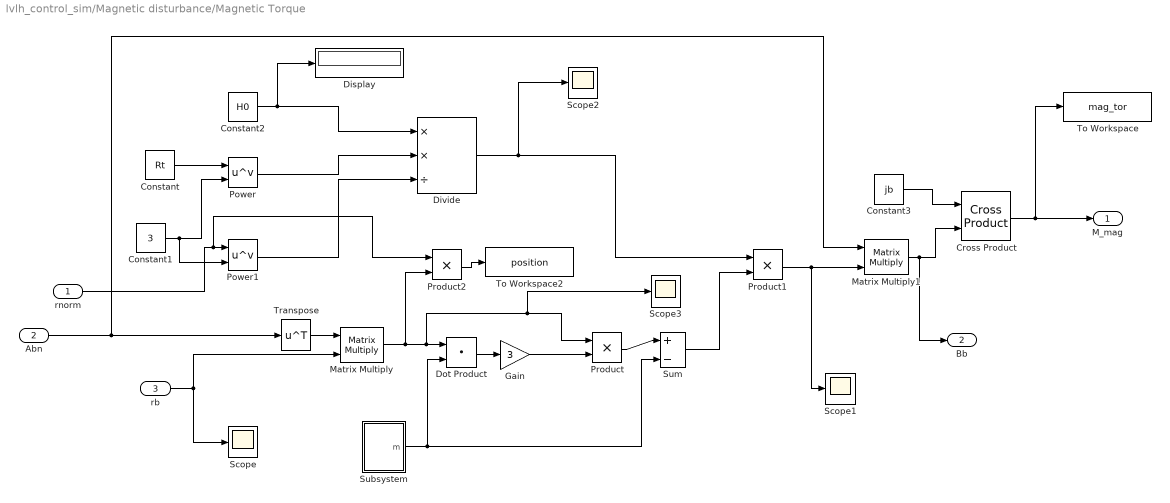
== system lvlh_control_sim/Magnetic disturbance/Magnetic Torque  ==
  rnorm : Inport
  Abn : Inport  Port=2
  rb : Inport  Port=3
  Constant : Constant  Value=Rt
  Constant1 : Constant  Value=3
  Constant2 : Constant  Value=H0
  Constant3 : Constant  Value=jb
  Cross Product : matrix_library/Cross Product
  Display : Display
  Divide : Product  Inputs=**/
  Dot Product : DotProduct  OutDataTypeStr=Inherit: Inherit via internal rule
  Gain : Gain  Gain=3
  Matrix Multiply : Product  Multiplication=Matrix(*)
  Matrix Multiply1 : Product  Multiplication=Matrix(*)
  Power : Math  Operator=pow
  Power1 : Math  Operator=pow
  Product : Product
  Product1 : Product
  Product2 : Product
  Scope{,1..3} (4 alike) : Scope
  Subsystem : Subsystem
  Sum : Sum  Inputs=|+-
  To Workspace : ToWorkspace  VariableName=mag_tor  SampleTime=-1
  To Workspace2 : ToWorkspace  VariableName=position  SampleTime=-1
  Transpose : Math  Operator=transpose
  M_mag : Outport
  Bb : Outport  Port=2
  wires:
  Abn/1 -> Matrix Multiply1/1, Transpose/1
  Transpose/1 -> Matrix Multiply/1
  rb/1 -> Scope/1, Matrix Multiply/2
  Matrix Multiply/1 -> Product2/2, Scope3/1, Product/1, Dot Product/1
  Subsystem/1(m) -> Sum/2, Dot Product/2
  Dot Product/1 -> Gain/1
  Gain/1 -> Product/2
  Product/1 -> Sum/1
  Constant/1 -> Power/1
  Constant1/1 -> Power1/2, Power/2
  rnorm/1 -> Product2/1, Power1/1
  Constant2/1 -> Display/1, Divide/1
  Power/1 -> Divide/2
  Power1/1 -> Divide/3
  Divide/1 -> Scope2/1, Product1/1
  Sum/1 -> Product1/2
  Product1/1 -> Scope1/1, Matrix Multiply1/2
  Constant3/1 -> Cross Product/1
  Matrix Multiply1/1 -> Bb/1, Cross Product/2
  Cross Product/1 -> To Workspace/1, M_mag/1
  Product2/1 -> To Workspace2/1

== system lvlh_control_sim/Sun Sensor/FOV CHECK ==
  In1 : Inport
  Acos : Trigonometry  Operator=acos
  Dot Product : DotProduct  OutDataTypeStr=Inherit: Inherit via internal rule
  FOV angle : Constant  Value=FOV_sun
  Less Than : RelationalOperator  Operator=<  OutDataTypeStr=boolean  RndMeth=Simplest  InputSameDT=off
  optical axis : Constant  Value=[0;0;1]
  b : Outport
  wires:
  optical axis/1 -> Dot Product/1
  In1/1 -> Dot Product/2
  Dot Product/1 -> Acos/1
  FOV angle/1 -> Less Than/2
  Acos/1 -> Less Than/1
  Less Than/1 -> b/1

== system lvlh_control_sim/Sun Sensor/Sun Sensor Modeling ==
  Sb : Inport
  Cross Product : matrix_library/Cross Product
  Normalization1 : dspmathops/Normalization  NormType=2-norm  Bias=1e-10  NormOver=Each column  Dimension=1  roundingMode=Floor  overflowMode=off  accumDataTypeStr=Inherit: Same as product output  accumLastDataTypeStr=Inherit: Same as product output  outputDataTypeStr=Inherit: Same as product output  outputMin=[]  outputMax=[]  outputLastDataTypeStr=Inherit: Same as product output
  Normalize Vector : vrlib/Utilities/Normalize Vector  maxzero=0
  Product : Product
  Random Number : RandomNumber  Variance=tan(deg2rad(1/60))^2  SampleTime=1/freq_sun
  Sum2 : Sum
  Uniform Random Number : UniformRandomNumber  SampleTime=1/freq_sun
  Uniform Random Number1 : UniformRandomNumber  SampleTime=1/freq_sun
  Uniform Random Number2 : UniformRandomNumber  SampleTime=1/freq_sun
  Vector Concatenate : Concatenate  NumInputs=3
  Zero-Order Hold : ZeroOrderHold  SampleTime=1/freq_sun
  s3 : Outport
  wires:
  Zero-Order Hold/1 -> Cross Product/2, Sum2/2  "Sb"
  Cross Product/1 -> Normalization1/1
  Sum2/1 -> Normalize Vector/1  "q"
  Uniform Random Number1/1 -> Vector Concatenate/2
  Vector Concatenate/1 -> Cross Product/1
  Normalization1/1 -> Product/2
  Uniform Random Number2/1 -> Vector Concatenate/3
  Normalize Vector/1 -> s3/1
  Uniform Random Number/1 -> Vector Concatenate/1
  Product/1 -> Sum2/1
  Random Number/1 -> Product/1
  Sb/1 -> Zero-Order Hold/1

== system lvlh_control_sim/kep_dyn/r_norm ==
  e : Inport
  theta : Inport  Port=2
  Constant : Constant  Value=a
  Constant1 : Constant
  Cos : Trigonometry  Operator=cos
  Divide : Product  Inputs=*/
  Power : Math  Operator=magnitude^2
  Product : Product
  Product1 : Product
  Sum : Sum  Inputs=+-
  Sum2 : Sum
  r : Outport
  wires:
  e/1 -> Product1/2, Power/1
  Power/1 -> Sum/2
  Constant1/1 -> Sum2/2, Sum/1
  Sum/1 -> Product/2
  Constant/1 -> Product/1
  theta/1 -> Cos/1
  Cos/1 -> Product1/1
  Product1/1 -> Sum2/1
  Product/1 -> Divide/1
  Sum2/1 -> Divide/2
  Divide/1 -> r/1

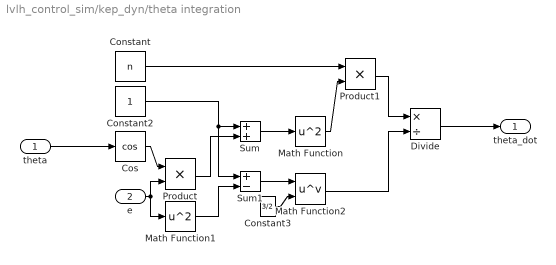
== system lvlh_control_sim/kep_dyn/theta integration ==
  theta : Inport
  e : Inport  Port=2
  Constant : Constant  Value=n
  Constant2 : Constant
  Constant3 : Constant  Value=3/2
  Cos : Trigonometry  Operator=cos
  Divide : Product  Inputs=*/
  Math Function : Math  Operator=square
  Math Function1 : Math  Operator=square
  Math Function2 : Math  Operator=pow
  Product : Product
  Product1 : Product
  Sum : Sum
  Sum1 : Sum  Inputs=+-
  theta_dot : Outport
  wires:
  Product1/1 -> Divide/1
  Product/1 -> Sum/2
  Math Function2/1 -> Divide/2
  Sum1/1 -> Math Function2/1
  Constant2/1 -> Sum1/1, Sum/1
  Math Function1/1 -> Sum1/2
  e/1 -> Product/2, Math Function1/1
  Constant3/1 -> Math Function2/2
  Constant/1 -> Product1/1
  Sum/1 -> Math Function/1
  Math Function/1 -> Product1/2
  Cos/1 -> Product/1
  theta/1 -> Cos/1
  Divide/1 -> theta_dot/1

== system lvlh_control_sim/relative kinematics/Subsystem ==
  theta : Inport
  Constant3 : Constant
  Constant4 : Constant  Value=0
  Cos2 : Trigonometry  Operator=cos
  Cos3 : Trigonometry
  Gain : Gain  Gain=-1
  Matrix Concatenate1 : Concatenate  NumInputs=3  Mode=Multidimensional array  ConcatenateDimension=2
  Vector Concatenate : Concatenate  NumInputs=3
  Vector Concatenate1 : Concatenate  NumInputs=3
  Vector Concatenate2 : Concatenate  NumInputs=3
  A_PL : Outport
  wires:
  Constant4/1 -> Vector Concatenate2/2, Vector Concatenate/3, Vector Concatenate1/3, Vector Concatenate2/1
  Vector Concatenate/1 -> Matrix Concatenate1/1
  Cos2/1 -> Vector Concatenate1/2, Vector Concatenate/1
  Gain/1 -> Vector Concatenate1/1
  Cos3/1 -> Vector Concatenate/2, Gain/1
  Constant3/1 -> Vector Concatenate2/3
  Vector Concatenate2/1 -> Matrix Concatenate1/3
  Vector Concatenate1/1 -> Matrix Concatenate1/2
  theta/1 -> Cos2/1, Cos3/1
  Matrix Concatenate1/1 -> A_PL/1  "A_PL"

== system lvlh_control_sim/Kinematics/Kinematics 312/A - s_312 ==
  A : Inport
  Asin : Trigonometry  Operator=asin
  Atan1 : Trigonometry  Operator=atan2
  Atan2 : Trigonometry  Operator=atan2
  Gain : Gain  Gain=-1
  Gain1 : Gain  Gain=-1
  Mux : Mux  Inputs=3
  Selector : Selector  NumberOfDimensions=2  InputPortWidth=3  IndexOptions=Index vector (dialog),Index vector (dialog)  Indices=2,1  OutputSizes=1,1
  Selector1 : Selector  NumberOfDimensions=2  InputPortWidth=3  IndexOptions=Index vector (dialog),Index vector (dialog)  Indices=2,2  OutputSizes=1,1
  Selector2 : Selector  NumberOfDimensions=2  InputPortWidth=3  IndexOptions=Index vector (dialog),Index vector (dialog)  Indices=2,3  OutputSizes=1,1
  Selector3 : Selector  NumberOfDimensions=2  InputPortWidth=3  IndexOptions=Index vector (dialog),Index vector (dialog)  Indices=1,3  OutputSizes=1,1
  Selector4 : Selector  NumberOfDimensions=2  InputPortWidth=3  IndexOptions=Index vector (dialog),Index vector (dialog)  Indices=3,3  OutputSizes=1,1
  s : Outport
  wires:
  Mux/1 -> s/1
  Selector4/1 -> Atan1/2  "a33"
  Atan1/1 -> Mux/3  "psi"
  Atan2/1 -> Mux/1  "phi"
  A/1 -> Selector2/1, Selector1/1, Selector/1, Selector3/1, Selector4/1
  Selector2/1 -> Asin/1  "a23"
  Selector3/1 -> Gain1/1  "a13"
  Selector1/1 -> Atan2/2  "a22"
  Selector/1 -> Gain/1  "a21"
  Asin/1 -> Mux/2  "theta"
  Gain/1 -> Atan2/1
  Gain1/1 -> Atan1/1

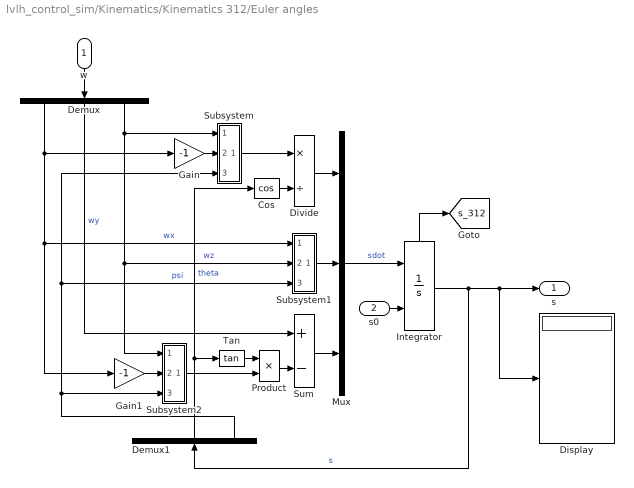
== system lvlh_control_sim/Kinematics/Kinematics 312/Euler angles ==
  w : Inport
  s0 : Inport  Port=2
  Cos : Trigonometry  Operator=cos
  Demux : Demux  Outputs=3
  Demux1 : Demux  Outputs=3
  Display : Display
  Divide : Product  Inputs=*/
  Gain : Gain  Gain=-1
  Gain1 : Gain  Gain=-1
  Integrator : Integrator  InitialConditionSource=external  InitialCondition=s0  WrapState=on  WrappedStateUpperValue=2*pi  WrappedStateLowerValue=0  ShowStatePort=on
  Mux : Mux  Inputs=3
  Product : Product
  Subsystem : Subsystem
  Subsystem1 : Subsystem
  Subsystem2 : Subsystem
  Sum : Sum  Inputs=+-
  Tan : Trigonometry  Operator=tan
  s : Outport
  tag scope: s_312=global
  wires:
  w/1 -> Demux/1
  Integrator/1 -> Demux1/1, Display/1, s/1  "s"
  Demux/3 -> Subsystem2/1(In1), Subsystem1/2(In2), Subsystem/1(In1)  "wz"
  Gain/1 -> Subsystem/2(In2)
  Demux/1 -> Gain1/1, Subsystem1/1(In1), Gain/1  "wx"
  Demux1/3 -> Subsystem2/3(In3), Subsystem1/3(In3), Subsystem/3(In3)  "psi"
  Subsystem/1(Out1) -> Divide/1
  Cos/1 -> Divide/2
  Demux1/2 -> Cos/1, Tan/1  "theta"
  Divide/1 -> Mux/1
  Subsystem1/1(Out1) -> Mux/2
  Gain1/1 -> Subsystem2/2(In2)
  Tan/1 -> Product/1
  Subsystem2/1(Out1) -> Product/2
  Product/1 -> Sum/2
  Demux/2 -> Sum/1  "wy"
  Sum/1 -> Mux/3
  Mux/1 -> Integrator/1  "sdot"
  s0/1 -> Integrator/2
  Integrator/State -> [s_312]

== system lvlh_control_sim/Kinematics/Kinematics 312/s_312 - A ==
  s : Inport
  Demux : Demux  Outputs=3
  Product : Product  Inputs=3  Multiplication=Matrix(*)
  R1 : Subsystem
  R2 : Subsystem
  R3 : Subsystem
  A : Outport
  wires:
  s/1 -> Demux/1  "s"
  R1/1(R1) -> Product/2
  R3/1(R3) -> Product/3
  R2/1(R2) -> Product/1
  Product/1 -> A/1
  Demux/2 -> R1/1(x)  "theta"
  Demux/1 -> R3/1(x)  "phi"
  Demux/3 -> R2/1(x)  "psi"

== system lvlh_control_sim/Kinematics/Kinematics 312/s_313 - A ==
  s : Inport
  Demux : Demux  Outputs=3
  Product : Product  Inputs=3  Multiplication=Matrix(*)
  R1 : Subsystem
  R3_1 : Subsystem
  R3_2 : Subsystem
  A : Outport
  wires:
  Demux/3 -> R3_2/1(x)  "psi"
  Demux/1 -> R3_1/1(x)  "phi"
  Demux/2 -> R1/1(x)  "theta"
  Product/1 -> A/1
  R1/1(R1) -> Product/2
  s/1 -> Demux/1  "s"
  R3_1/1(R3) -> Product/3
  R3_2/1(R3) -> Product/1

== system lvlh_control_sim/Kinematics/Kinematics 313/A - s_313 ==
  A : Inport
  Acos : Trigonometry  Operator=acos
  Atan1 : Trigonometry  Operator=atan2
  Atan2 : Trigonometry  Operator=atan2
  Gain : Gain  Gain=-1
  Mux : Mux  Inputs=3
  Selector : Selector  NumberOfDimensions=2  InputPortWidth=3  IndexOptions=Index vector (dialog),Index vector (dialog)  Indices=3,1  OutputSizes=1,1
  Selector1 : Selector  NumberOfDimensions=2  InputPortWidth=3  IndexOptions=Index vector (dialog),Index vector (dialog)  Indices=3,2  OutputSizes=1,1
  Selector2 : Selector  NumberOfDimensions=2  InputPortWidth=3  IndexOptions=Index vector (dialog),Index vector (dialog)  Indices=3,3  OutputSizes=1,1
  Selector3 : Selector  NumberOfDimensions=2  InputPortWidth=3  IndexOptions=Index vector (dialog),Index vector (dialog)  Indices=1,3  OutputSizes=1,1
  Selector4 : Selector  NumberOfDimensions=2  InputPortWidth=3  IndexOptions=Index vector (dialog),Index vector (dialog)  Indices=2,3  OutputSizes=1,1
  s : Outport
  wires:
  Acos/1 -> Mux/2  "theta"
  Selector/1 -> Atan2/1  "a31"
  Selector1/1 -> Gain/1  "a32"
  Selector3/1 -> Atan1/1  "a13"
  Selector2/1 -> Acos/1  "a33"
  A/1 -> Selector4/1, Selector3/1, Selector/1, Selector1/1, Selector2/1
  Atan2/1 -> Mux/1  "phi"
  Atan1/1 -> Mux/3  "psi"
  Gain/1 -> Atan2/2
  Selector4/1 -> Atan1/2  "a23"
  Mux/1 -> s/1

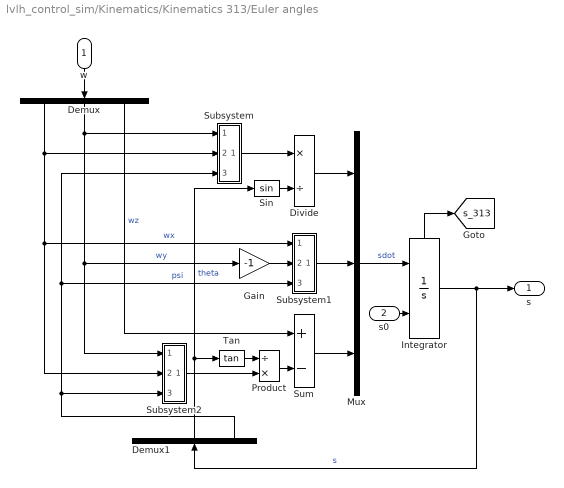
== system lvlh_control_sim/Kinematics/Kinematics 313/Euler angles ==
  w : Inport
  s0 : Inport  Port=2
  Demux : Demux  Outputs=3
  Demux1 : Demux  Outputs=3
  Divide : Product  Inputs=*/
  Gain : Gain  Gain=-1
  Integrator : Integrator  InitialConditionSource=external  InitialCondition=s0  WrapState=on  WrappedStateUpperValue=2*pi  WrappedStateLowerValue=0  ShowStatePort=on
  Mux : Mux  Inputs=3
  Product : Product  Inputs=/*
  Sin : Trigonometry
  Subsystem : Subsystem
  Subsystem1 : Subsystem
  Subsystem2 : Subsystem
  Sum : Sum  Inputs=+-
  Tan : Trigonometry  Operator=tan
  s : Outport
  tag scope: s_313=global
  wires:
  Mux/1 -> Integrator/1  "sdot"
  Sum/1 -> Mux/3
  Demux/2 -> Subsystem/1(In1), Subsystem2/1(In1), Gain/1  "wy"
  Product/1 -> Sum/2
  Subsystem2/1(Out1) -> Product/2
  Tan/1 -> Product/1
  Subsystem1/1(Out1) -> Mux/2
  Divide/1 -> Mux/1
  Demux1/2 -> Sin/1, Tan/1  "theta"
  Subsystem/1(Out1) -> Divide/1
  Demux1/3 -> Subsystem/3(In3), Subsystem1/3(In3), Subsystem2/3(In3)  "psi"
  Demux/1 -> Subsystem2/2(In2), Subsystem1/1(In1), Subsystem/2(In2)  "wx"
  Demux/3 -> Sum/1  "wz"
  Integrator/1 -> Demux1/1, s/1  "s"
  w/1 -> Demux/1
  Sin/1 -> Divide/2
  Gain/1 -> Subsystem1/2(In2)
  s0/1 -> Integrator/2
  Integrator/State -> [s_313]

== system lvlh_control_sim/Kinematics/Kinematics 313/s_312 - A ==
  s : Inport
  Demux : Demux  Outputs=3
  Product : Product  Inputs=3  Multiplication=Matrix(*)
  R1 : Subsystem
  R2 : Subsystem
  R3 : Subsystem
  A : Outport
  wires:
  s/1 -> Demux/1  "s"
  R1/1(R1) -> Product/2
  R3/1(R3) -> Product/3
  R2/1(R2) -> Product/1
  Product/1 -> A/1
  Demux/2 -> R1/1(x)  "theta"
  Demux/1 -> R3/1(x)  "phi"
  Demux/3 -> R2/1(x)  "psi"

== system lvlh_control_sim/Kinematics/Kinematics 313/s_313 - A ==
  s : Inport
  Demux : Demux  Outputs=3
  Product : Product  Inputs=3  Multiplication=Matrix(*)
  R1 : Subsystem
  R3_1 : Subsystem
  R3_2 : Subsystem
  A : Outport
  wires:
  Demux/3 -> R3_2/1(x)  "psi"
  Demux/1 -> R3_1/1(x)  "phi"
  Demux/2 -> R1/1(x)  "theta"
  Product/1 -> A/1
  R1/1(R1) -> Product/2
  s/1 -> Demux/1  "s"
  R3_1/1(R3) -> Product/3
  R3_2/1(R3) -> Product/1

== system lvlh_control_sim/Magnetic disturbance/Magnetic Torque /Subsystem ==
  Clock : Clock
  Constant : Constant  Value=incl
  Constant1 : Constant  Value=omegaE
  Cos : Trigonometry  Operator=cos
  Cos1 : Trigonometry  Operator=cos
  Product : Product
  Product1 : Product
  Product2 : Product
  Scope : Scope
  Sin : Trigonometry
  Sin1 : Trigonometry
  Vector Concatenate : Concatenate  NumInputs=3
  m : Outport
  wires:
  Constant/1 -> Cos/1, Sin/1
  Clock/1 -> Product/1
  Constant1/1 -> Product/2
  Product/1 -> Sin1/1, Cos1/1
  Cos1/1 -> Product1/1
  Sin/1 -> Product2/2, Product1/2
  Sin1/1 -> Product2/1
  Product1/1 -> Vector Concatenate/1
  Product2/1 -> Vector Concatenate/2
  Cos/1 -> Vector Concatenate/3
  Vector Concatenate/1 -> Scope/1, m/1

== system lvlh_control_sim/Kinematics/Kinematics 312/Euler angles/Subsystem ==
  In1 : Inport
  In2 : Inport  Port=2
  In3 : Inport  Port=3
  Cos : Trigonometry  Operator=cos
  Product : Product
  Product1 : Product
  Sin : Trigonometry
  Sum : Sum
  Out1 : Outport
  wires:
  In3/1 -> Sin/1, Cos/1
  In1/1 -> Product/1
  Cos/1 -> Product/2
  Sin/1 -> Product1/1
  In2/1 -> Product1/2
  Product/1 -> Sum/1
  Product1/1 -> Sum/2
  Sum/1 -> Out1/1

== system lvlh_control_sim/Kinematics/Kinematics 312/Euler angles/Subsystem1 ==
  In1 : Inport
  In2 : Inport  Port=2
  In3 : Inport  Port=3
  Cos : Trigonometry  Operator=cos
  Product : Product
  Product1 : Product
  Sin : Trigonometry
  Sum : Sum
  Out1 : Outport
  wires:
  Sum/1 -> Out1/1
  Product1/1 -> Sum/2
  Product/1 -> Sum/1
  In2/1 -> Product1/2
  Sin/1 -> Product1/1
  Cos/1 -> Product/2
  In1/1 -> Product/1
  In3/1 -> Cos/1, Sin/1

== system lvlh_control_sim/Kinematics/Kinematics 312/Euler angles/Subsystem2 ==
  In1 : Inport
  In2 : Inport  Port=2
  In3 : Inport  Port=3
  Cos : Trigonometry  Operator=cos
  Product : Product
  Product1 : Product
  Sin : Trigonometry
  Sum : Sum
  Out1 : Outport
  wires:
  In3/1 -> Sin/1, Cos/1
  In1/1 -> Product/1
  Cos/1 -> Product/2
  Sin/1 -> Product1/1
  In2/1 -> Product1/2
  Product/1 -> Sum/1
  Product1/1 -> Sum/2
  Sum/1 -> Out1/1

== system lvlh_control_sim/Kinematics/Kinematics 312/s_312 - A/R1 ==
  x : Inport
  Constant : Constant  Value=[1; 0; 0]
  Constant1 : Constant  Value=0
  Cos : Trigonometry  Operator=cos
  Gain : Gain  Gain=-1
  Matrix Concatenate : Concatenate  NumInputs=3  Mode=Multidimensional array  ConcatenateDimension=2
  Sin : Trigonometry
  Vector Concatenate : Concatenate  NumInputs=3
  Vector Concatenate1 : Concatenate  NumInputs=3
  R1 : Outport
  wires:
  Matrix Concatenate/1 -> R1/1
  x/1 -> Cos/1, Sin/1
  Vector Concatenate1/1 -> Matrix Concatenate/2
  Constant/1 -> Matrix Concatenate/1
  Vector Concatenate/1 -> Matrix Concatenate/3
  Constant1/1 -> Vector Concatenate/1, Vector Concatenate1/1
  Cos/1 -> Vector Concatenate/3, Vector Concatenate1/2
  Gain/1 -> Vector Concatenate1/3
  Sin/1 -> Vector Concatenate/2, Gain/1

== system lvlh_control_sim/Kinematics/Kinematics 312/s_312 - A/R2 ==
  x : Inport
  Constant : Constant  Value=[0; 1; 0]
  Constant1 : Constant  Value=0
  Cos : Trigonometry  Operator=cos
  Gain : Gain  Gain=-1
  Matrix Concatenate : Concatenate  NumInputs=3  Mode=Multidimensional array  ConcatenateDimension=2
  Sin : Trigonometry
  Vector Concatenate : Concatenate  NumInputs=3
  Vector Concatenate1 : Concatenate  NumInputs=3
  R2 : Outport
  wires:
  Vector Concatenate/1 -> Matrix Concatenate/1
  x/1 -> Sin/1, Cos/1
  Matrix Concatenate/1 -> R2/1
  Constant/1 -> Matrix Concatenate/2
  Vector Concatenate1/1 -> Matrix Concatenate/3
  Constant1/1 -> Vector Concatenate/2, Vector Concatenate1/2
  Cos/1 -> Vector Concatenate1/3, Vector Concatenate/1
  Sin/1 -> Gain/1, Vector Concatenate/3
  Gain/1 -> Vector Concatenate1/1

== system lvlh_control_sim/Kinematics/Kinematics 312/s_312 - A/R3 ==
  x : Inport
  Constant : Constant  Value=[0; 0; 1]
  Constant1 : Constant  Value=0
  Cos : Trigonometry  Operator=cos
  Gain : Gain  Gain=-1
  Matrix Concatenate : Concatenate  NumInputs=3  Mode=Multidimensional array  ConcatenateDimension=2
  Sin : Trigonometry
  Vector Concatenate : Concatenate  NumInputs=3
  Vector Concatenate1 : Concatenate  NumInputs=3
  R3 : Outport
  wires:
  Vector Concatenate/1 -> Matrix Concatenate/1
  Sin/1 -> Vector Concatenate1/1, Gain/1
  Cos/1 -> Vector Concatenate1/2, Vector Concatenate/1
  Constant/1 -> Matrix Concatenate/3
  Gain/1 -> Vector Concatenate/2
  Vector Concatenate1/1 -> Matrix Concatenate/2
  x/1 -> Sin/1, Cos/1
  Constant1/1 -> Vector Concatenate/3, Vector Concatenate1/3
  Matrix Concatenate/1 -> R3/1

== system lvlh_control_sim/Kinematics/Kinematics 312/s_313 - A/R1 ==
  x : Inport
  Constant : Constant  Value=[1; 0; 0]
  Constant1 : Constant  Value=0
  Cos : Trigonometry  Operator=cos
  Gain : Gain  Gain=-1
  Matrix Concatenate : Concatenate  NumInputs=3  Mode=Multidimensional array  ConcatenateDimension=2
  Sin : Trigonometry
  Vector Concatenate : Concatenate  NumInputs=3
  Vector Concatenate1 : Concatenate  NumInputs=3
  R1 : Outport
  wires:
  Sin/1 -> Gain/1, Vector Concatenate/2
  Gain/1 -> Vector Concatenate1/3
  Cos/1 -> Vector Concatenate1/2, Vector Concatenate/3
  Constant1/1 -> Vector Concatenate1/1, Vector Concatenate/1
  Vector Concatenate/1 -> Matrix Concatenate/3
  Constant/1 -> Matrix Concatenate/1
  Vector Concatenate1/1 -> Matrix Concatenate/2
  x/1 -> Sin/1, Cos/1
  Matrix Concatenate/1 -> R1/1

== system lvlh_control_sim/Kinematics/Kinematics 312/s_313 - A/R3_1 ==
  x : Inport
  Constant : Constant  Value=[0; 0; 1]
  Constant1 : Constant  Value=0
  Cos : Trigonometry  Operator=cos
  Gain : Gain  Gain=-1
  Matrix Concatenate : Concatenate  NumInputs=3  Mode=Multidimensional array  ConcatenateDimension=2
  Sin : Trigonometry
  Vector Concatenate : Concatenate  NumInputs=3
  Vector Concatenate1 : Concatenate  NumInputs=3
  R3 : Outport
  wires:
  Matrix Concatenate/1 -> R3/1
  Constant1/1 -> Vector Concatenate1/3, Vector Concatenate/3
  x/1 -> Cos/1, Sin/1
  Vector Concatenate1/1 -> Matrix Concatenate/2
  Gain/1 -> Vector Concatenate/2
  Constant/1 -> Matrix Concatenate/3
  Cos/1 -> Vector Concatenate/1, Vector Concatenate1/2
  Sin/1 -> Gain/1, Vector Concatenate1/1
  Vector Concatenate/1 -> Matrix Concatenate/1

== system lvlh_control_sim/Kinematics/Kinematics 312/s_313 - A/R3_2 ==
  x : Inport
  Constant : Constant  Value=[0; 0; 1]
  Constant1 : Constant  Value=0
  Cos : Trigonometry  Operator=cos
  Gain : Gain  Gain=-1
  Matrix Concatenate : Concatenate  NumInputs=3  Mode=Multidimensional array  ConcatenateDimension=2
  Sin : Trigonometry
  Vector Concatenate : Concatenate  NumInputs=3
  Vector Concatenate1 : Concatenate  NumInputs=3
  R3 : Outport
  wires:
  Vector Concatenate/1 -> Matrix Concatenate/1
  Sin/1 -> Vector Concatenate1/1, Gain/1
  Cos/1 -> Vector Concatenate1/2, Vector Concatenate/1
  Constant/1 -> Matrix Concatenate/3
  Gain/1 -> Vector Concatenate/2
  Vector Concatenate1/1 -> Matrix Concatenate/2
  x/1 -> Sin/1, Cos/1
  Constant1/1 -> Vector Concatenate/3, Vector Concatenate1/3
  Matrix Concatenate/1 -> R3/1

== system lvlh_control_sim/Kinematics/Kinematics 313/Euler angles/Subsystem ==
  In1 : Inport
  In2 : Inport  Port=2
  In3 : Inport  Port=3
  Cos : Trigonometry  Operator=cos
  Product : Product
  Product1 : Product
  Sin : Trigonometry
  Sum : Sum
  Out1 : Outport
  wires:
  Sum/1 -> Out1/1
  Product1/1 -> Sum/2
  Product/1 -> Sum/1
  In2/1 -> Product1/2
  Sin/1 -> Product1/1
  Cos/1 -> Product/2
  In1/1 -> Product/1
  In3/1 -> Cos/1, Sin/1

== system lvlh_control_sim/Kinematics/Kinematics 313/Euler angles/Subsystem1 ==
  In1 : Inport
  In2 : Inport  Port=2
  In3 : Inport  Port=3
  Cos : Trigonometry  Operator=cos
  Product : Product
  Product1 : Product
  Sin : Trigonometry
  Sum : Sum
  Out1 : Outport
  wires:
  In3/1 -> Sin/1, Cos/1
  In1/1 -> Product/1
  Cos/1 -> Product/2
  Sin/1 -> Product1/1
  In2/1 -> Product1/2
  Product/1 -> Sum/1
  Product1/1 -> Sum/2
  Sum/1 -> Out1/1

== system lvlh_control_sim/Kinematics/Kinematics 313/Euler angles/Subsystem2 ==
  In1 : Inport
  In2 : Inport  Port=2
  In3 : Inport  Port=3
  Cos : Trigonometry  Operator=cos
  Product : Product
  Product1 : Product
  Sin : Trigonometry
  Sum : Sum
  Out1 : Outport
  wires:
  Sum/1 -> Out1/1
  Product1/1 -> Sum/2
  Product/1 -> Sum/1
  In2/1 -> Product1/2
  Sin/1 -> Product1/1
  Cos/1 -> Product/2
  In1/1 -> Product/1
  In3/1 -> Cos/1, Sin/1
